simulink model "DCMotor"  (Simulink 7.9)
settings: Solver=ode3  StartTime=0.0  StopTime=50  FixedStep=100e-6  RelTol=1e-3
settings Model: Creator=Dionis  LastModifiedBy=dep02378
settings OptimizationCC: ExpressionDepthLimit=128
settings DebuggingCC: MultiTaskDSMMsg=warning  MultiTaskCondExecSysMsg=none  StateNameClashWarn=none  StrictBusMsg=None
settings RTWCC: IncludeERTFirstTime=on
settings CodeAppCC: CustomSymbolStrType=$N$R$M_T

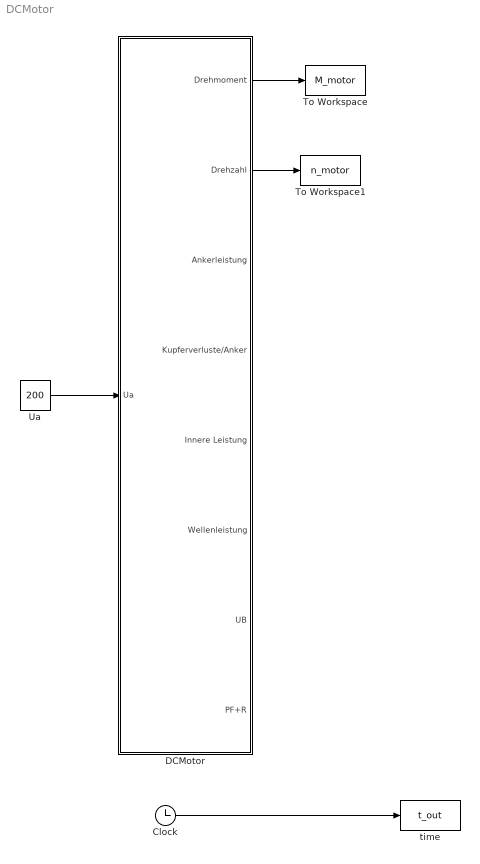
== system DCMotor ==
  Clock : Clock
  DCMotor : Subsystem
  To Workspace : ToWorkspace  VariableName=M_motor  SampleTime=-1
  To Workspace1 : ToWorkspace  VariableName=n_motor  SampleTime=-1
  Ua : Constant  Value=200
  time : ToWorkspace  VariableName=t_out  SampleTime=-1
  wires:
  Ua/1 -> DCMotor/1(Ua)
  DCMotor/1(Drehmoment) -> To Workspace/1
  Clock/1 -> time/1
  DCMotor/2(Drehzahl) -> To Workspace1/1

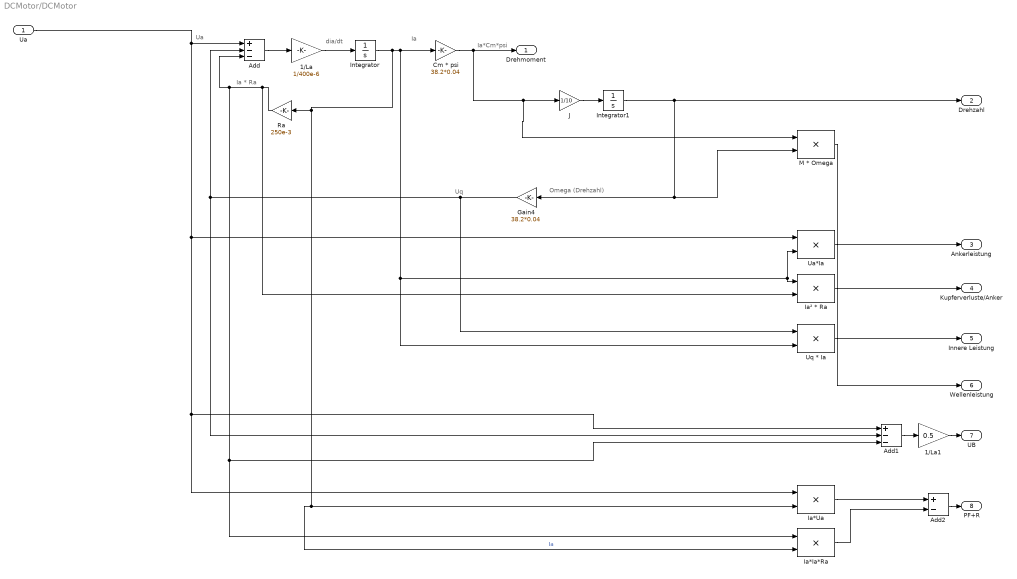
== system DCMotor/DCMotor ==
  note: Ua
  note: Omega (Drehzahl)
  note: Uq
  note: Ia*Cm*psi
  note: Ia * Ra
  note: Ia
  note: dia/dt
  Ua : Inport
  1/La : Gain  Gain=1/400e-6
  1/La1 : Gain  Gain=0.5
  Add : Sum  Inputs=+--
  Add1 : Sum  Inputs=+--
  Add2 : Sum  Inputs=+-
  Cm * psi : Gain  Gain=38.2*0.04
  Gain4 : Gain  Gain=38.2*0.04
  Ia*Ia*Ra : Product
  Ia*Ua : Product
  Ia² * Ra : Product
  Integrator : Integrator
  Integrator1 : Integrator
  J : Gain  Gain=1/10
  M * Omega : Product
  Ra : Gain  Gain=250e-3
  Ua*Ia : Product
  Uq * Ia : Product
  Drehmoment : Outport
  Drehzahl : Outport  Port=2
  Ankerleistung : Outport  Port=3
  Kupferverluste/Anker : Outport  Port=4
  Innere Leistung : Outport  Port=5
  Wellenleistung : Outport  Port=6
  UB : Outport  Port=7
  PF+R : Outport  Port=8
  wires:
  Ua/1 -> Add/1, Ua*Ia/1, Ia*Ua/1, Add1/1
  1/La/1 -> Integrator/1
  Integrator/1 -> Ua*Ia/2, Ia² * Ra/1, Uq * Ia/2, Cm * psi/1, Ia*Ua/2, Ia*Ia*Ra/2, Ra/1  "Ia"
  Add/1 -> 1/La/1
  Gain4/1 -> Add1/2, Add/2, Uq * Ia/1
  Uq * Ia/1 -> Innere Leistung/1
  Ia² * Ra/1 -> Kupferverluste/Anker/1
  Ua*Ia/1 -> Ankerleistung/1
  M * Omega/1 -> Wellenleistung/1
  Cm * psi/1 -> J/1, M * Omega/1, Drehmoment/1
  J/1 -> Integrator1/1
  1/La1/1 -> UB/1
  Add1/1 -> 1/La1/1
  Ra/1 -> Ia² * Ra/2, Ia*Ia*Ra/1, Add1/3, Add/3
  Ia*Ua/1 -> Add2/1
  Ia*Ia*Ra/1 -> Add2/2
  Add2/1 -> PF+R/1
  Integrator1/1 -> M * Omega/2, Gain4/1, Drehzahl/1
